simulink model "ForwardDyn_CTC_SCARA"  (R2023a)
settings: Solver=FixedStepAuto  StartTime=0.0  StopTime=10  FixedStep=0.01  RelTol=1e-3
libraries: slpidlib x4
settings Model: Creator=abdom  LastModifiedBy=abdom

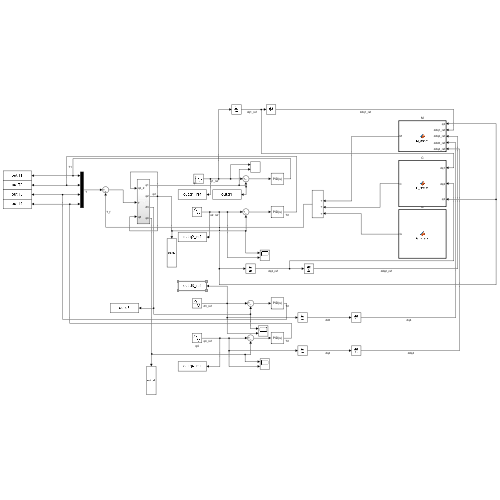
[thumbnail: Simulink's stored preview of the top-level diagram]
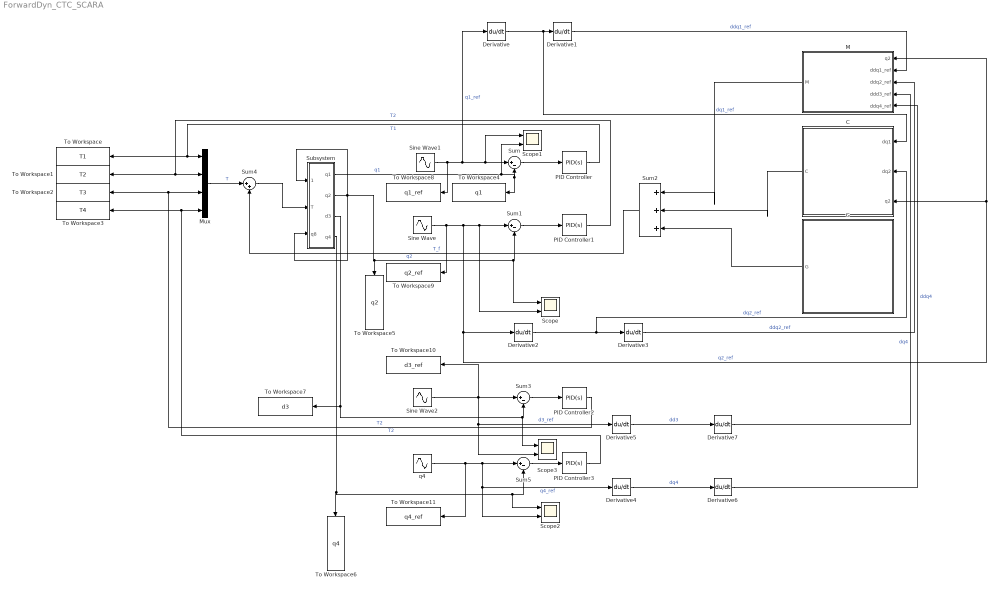
== system ForwardDyn_CTC_SCARA ==
  C : MATLAB Function  TreatAsAtomicUnit=on
  Derivative{,1..7} (8 alike) : Derivative
  G : MATLAB Function  TreatAsAtomicUnit=on
  M : MATLAB Function  TreatAsAtomicUnit=on
  Mux : Mux
  PID Controller : slpidlib/PID Controller  Controller=PID  Form=Parallel  TimeDomain=Continuous-time  UseExternalTs=off  SampleTime=-1  IntegratorMethod=Forward Euler  FilterMethod=Forward Euler  ControllerParametersSource=internal  P=100  I=70  UseKiTs=off  D=10  N=100  UseFilter=on  TunerSelectOption=Transfer Function Based (PID Tuner App)  InitialConditionSource=internal  InitialConditionForIntegrator=0  InitialConditionForFilter=0  DifferentiatorICPrevScaledInput=0  ExternalReset=none  TrackingMode=off  Kt=1  LimitOutput=off  SatLimitsSource=internal  UpperSaturationLimit=inf  LowerSaturationLimit=-inf  LinearizeAsGain=on  AntiWindupMode=none  Kb=1  LimitIntegrator=off  UpperIntegratorSaturationLimit=inf  LowerIntegratorSaturationLimit=-inf  POutMin=[]  POutMax=[]  IOutMin=[]  IOutMax=[]  DOutMin=[]  DOutMax=[]  NOutMin=[]  NOutMax=[]  SumOutMin=[]  SumOutMax=[]  SaturationOutMin=[]  SaturationOutMax=[]  PParamMin=[]  PParamMax=[]  IParamMin=[]  IParamMax=[]  DParamMin=[]  DParamMax=[]  NParamMin=[]  NParamMax=[]  KbParamMin=[]  KbParamMax=[]  KtParamMin=[]  KtParamMax=[]  KbOutMin=[]  KbOutMax=[]  KtOutMin=[]  KtOutMax=[]  IntegratorOutMin=[]  IntegratorOutMax=[]  FilterOutMin=[]  FilterOutMax=[]  SumI1OutMin=[]  SumI1OutMax=[]  SumI2OutMin=[]  SumI2OutMax=[]  SumI3OutMin=[]  SumI3OutMax=[]  SumI4OutMin=[]  SumI4OutMax=[]  SumDOutMin=[]  SumDOutMax=[]  DifferentiatorOutMin=[]  DifferentiatorOutMax=[]  FilterDiffOutCoefMin=[]  FilterDiffOutCoefMax=[]  ReciprocalOutMin=[]  ReciprocalOutMax=[]  SumDenOutMin=[]  SumDenOutMax=[]  SumNumOutMin=[]  SumNumOutMax=[]  DivideOutMin=[]  DivideOutMax=[]  UdiffTsProdOutMin=[]  UdiffTsProdOutMax=[]  NTsProdOutMin=[]  NTsProdOutMax=[]  UintegralTsProdOutMin=[]  UintegralTsProdOutMax=[]  UngainTsProdOutMin=[]  UngainTsProdOutMax=[]  ClampingZeroOutDataTypeStr=Inherit: Inherit via back propagation  ClampingZeroOutMin=[]  ClampingZeroOutMax=[]  FilterDenConstantOutDataTypeStr=Inherit: Inherit via back propagation  FilterDenConstantOutMin=[]  FilterDenConstantOutMax=[]  PCopyOutDataTypeStr=Inherit: Inherit via back propagation  PCopyOutMin=[]  PCopyOutMax=[]  NCopyOutDataTypeStr=Inherit: Inherit via back propagation  NCopyOutMin=[]  NCopyOutMax=[]  IntegratorContinuousStateAttributes=''  IntegratorStateMustResolveToSignalObject=off  IntegratorRTWStateStorageClass=Auto  FilterContinuousStateAttributes=''  FilterStateMustResolveToSignalObject=off  FilterRTWStateStorageClass=Auto  ParallelPVariant=InternalParameters  IdealPVariant=Disabled  IVariant=InternalParameters  DVariant=InternalParameters  IntegratorVariant=Continuous  SatVariant=Disabled  AWVariant=Passthrough  PCopyVariant=Disabled  TRVariant=Disabled  FdbkBlocksVariant=Forward  IdealPFdbkVariant=Disabled  SatFdbkVariant=Disabled  DerivativeFilterVariant=ContFilter  NVariant=InternalParameters  NCopyVariant=Disabled  FilterICVariant=InternalICsFilter  IntegratorICVariant=InternalICs  ExternalResetVariant=Disabled  TRSumVariant=Passthrough  SumFdbkVariant=Disabled  SumVariant=Sum_PID  TsampFilterVariant=InternalTs  TsampNgainVariant=Passthrough  TsampIntegralVariant=Disabled_SignalSpec  ExternalSaturationOutDataTypeStr=Inherit: Same as second input
  PID Controller1 : slpidlib/PID Controller  Controller=PID  Form=Parallel  TimeDomain=Continuous-time  UseExternalTs=off  SampleTime=-1  IntegratorMethod=Forward Euler  FilterMethod=Forward Euler  ControllerParametersSource=internal  P=100  I=30  UseKiTs=off  D=10  N=1  UseFilter=on  TunerSelectOption=Transfer Function Based (PID Tuner App)  InitialConditionSource=internal  InitialConditionForIntegrator=0  InitialConditionForFilter=0  DifferentiatorICPrevScaledInput=0  ExternalReset=none  TrackingMode=off  Kt=1  LimitOutput=off  SatLimitsSource=internal  UpperSaturationLimit=inf  LowerSaturationLimit=-inf  LinearizeAsGain=on  AntiWindupMode=none  Kb=1  LimitIntegrator=off  UpperIntegratorSaturationLimit=inf  LowerIntegratorSaturationLimit=-inf  POutMin=[]  POutMax=[]  IOutMin=[]  IOutMax=[]  DOutMin=[]  DOutMax=[]  NOutMin=[]  NOutMax=[]  SumOutMin=[]  SumOutMax=[]  SaturationOutMin=[]  SaturationOutMax=[]  PParamMin=[]  PParamMax=[]  IParamMin=[]  IParamMax=[]  DParamMin=[]  DParamMax=[]  NParamMin=[]  NParamMax=[]  KbParamMin=[]  KbParamMax=[]  KtParamMin=[]  KtParamMax=[]  KbOutMin=[]  KbOutMax=[]  KtOutMin=[]  KtOutMax=[]  IntegratorOutMin=[]  IntegratorOutMax=[]  FilterOutMin=[]  FilterOutMax=[]  SumI1OutMin=[]  SumI1OutMax=[]  SumI2OutMin=[]  SumI2OutMax=[]  SumI3OutMin=[]  SumI3OutMax=[]  SumI4OutMin=[]  SumI4OutMax=[]  SumDOutMin=[]  SumDOutMax=[]  DifferentiatorOutMin=[]  DifferentiatorOutMax=[]  FilterDiffOutCoefMin=[]  FilterDiffOutCoefMax=[]  ReciprocalOutMin=[]  ReciprocalOutMax=[]  SumDenOutMin=[]  SumDenOutMax=[]  SumNumOutMin=[]  SumNumOutMax=[]  DivideOutMin=[]  DivideOutMax=[]  UdiffTsProdOutMin=[]  UdiffTsProdOutMax=[]  NTsProdOutMin=[]  NTsProdOutMax=[]  UintegralTsProdOutMin=[]  UintegralTsProdOutMax=[]  UngainTsProdOutMin=[]  UngainTsProdOutMax=[]  ClampingZeroOutDataTypeStr=Inherit: Inherit via back propagation  ClampingZeroOutMin=[]  ClampingZeroOutMax=[]  FilterDenConstantOutDataTypeStr=Inherit: Inherit via back propagation  FilterDenConstantOutMin=[]  FilterDenConstantOutMax=[]  PCopyOutDataTypeStr=Inherit: Inherit via back propagation  PCopyOutMin=[]  PCopyOutMax=[]  NCopyOutDataTypeStr=Inherit: Inherit via back propagation  NCopyOutMin=[]  NCopyOutMax=[]  IntegratorContinuousStateAttributes=''  IntegratorStateMustResolveToSignalObject=off  IntegratorRTWStateStorageClass=Auto  FilterContinuousStateAttributes=''  FilterStateMustResolveToSignalObject=off  FilterRTWStateStorageClass=Auto  ParallelPVariant=InternalParameters  IdealPVariant=Disabled  IVariant=InternalParameters  DVariant=InternalParameters  IntegratorVariant=Continuous  SatVariant=Disabled  AWVariant=Passthrough  PCopyVariant=Disabled  TRVariant=Disabled  FdbkBlocksVariant=Forward  IdealPFdbkVariant=Disabled  SatFdbkVariant=Disabled  DerivativeFilterVariant=ContFilter  NVariant=InternalParameters  NCopyVariant=Disabled  FilterICVariant=InternalICsFilter  IntegratorICVariant=InternalICs  ExternalResetVariant=Disabled  TRSumVariant=Passthrough  SumFdbkVariant=Disabled  SumVariant=Sum_PID  TsampFilterVariant=InternalTs  TsampNgainVariant=Passthrough  TsampIntegralVariant=Disabled_SignalSpec  ExternalSaturationOutDataTypeStr=Inherit: Same as second input
  PID Controller2 : slpidlib/PID Controller  Controller=PID  Form=Parallel  TimeDomain=Continuous-time  UseExternalTs=off  SampleTime=-1  IntegratorMethod=Forward Euler  FilterMethod=Forward Euler  ControllerParametersSource=internal  P=150  I=50  UseKiTs=off  D=5  N=1  UseFilter=on  TunerSelectOption=Transfer Function Based (PID Tuner App)  InitialConditionSource=internal  InitialConditionForIntegrator=0  InitialConditionForFilter=0  DifferentiatorICPrevScaledInput=0  ExternalReset=none  TrackingMode=off  Kt=1  LimitOutput=off  SatLimitsSource=internal  UpperSaturationLimit=inf  LowerSaturationLimit=-inf  LinearizeAsGain=on  AntiWindupMode=none  Kb=1  LimitIntegrator=off  UpperIntegratorSaturationLimit=inf  LowerIntegratorSaturationLimit=-inf  POutMin=[]  POutMax=[]  IOutMin=[]  IOutMax=[]  DOutMin=[]  DOutMax=[]  NOutMin=[]  NOutMax=[]  SumOutMin=[]  SumOutMax=[]  SaturationOutMin=[]  SaturationOutMax=[]  PParamMin=[]  PParamMax=[]  IParamMin=[]  IParamMax=[]  DParamMin=[]  DParamMax=[]  NParamMin=[]  NParamMax=[]  KbParamMin=[]  KbParamMax=[]  KtParamMin=[]  KtParamMax=[]  KbOutMin=[]  KbOutMax=[]  KtOutMin=[]  KtOutMax=[]  IntegratorOutMin=[]  IntegratorOutMax=[]  FilterOutMin=[]  FilterOutMax=[]  SumI1OutMin=[]  SumI1OutMax=[]  SumI2OutMin=[]  SumI2OutMax=[]  SumI3OutMin=[]  SumI3OutMax=[]  SumI4OutMin=[]  SumI4OutMax=[]  SumDOutMin=[]  SumDOutMax=[]  DifferentiatorOutMin=[]  DifferentiatorOutMax=[]  FilterDiffOutCoefMin=[]  FilterDiffOutCoefMax=[]  ReciprocalOutMin=[]  ReciprocalOutMax=[]  SumDenOutMin=[]  SumDenOutMax=[]  SumNumOutMin=[]  SumNumOutMax=[]  DivideOutMin=[]  DivideOutMax=[]  UdiffTsProdOutMin=[]  UdiffTsProdOutMax=[]  NTsProdOutMin=[]  NTsProdOutMax=[]  UintegralTsProdOutMin=[]  UintegralTsProdOutMax=[]  UngainTsProdOutMin=[]  UngainTsProdOutMax=[]  ClampingZeroOutDataTypeStr=Inherit: Inherit via back propagation  ClampingZeroOutMin=[]  ClampingZeroOutMax=[]  FilterDenConstantOutDataTypeStr=Inherit: Inherit via back propagation  FilterDenConstantOutMin=[]  FilterDenConstantOutMax=[]  PCopyOutDataTypeStr=Inherit: Inherit via back propagation  PCopyOutMin=[]  PCopyOutMax=[]  NCopyOutDataTypeStr=Inherit: Inherit via back propagation  NCopyOutMin=[]  NCopyOutMax=[]  IntegratorContinuousStateAttributes=''  IntegratorStateMustResolveToSignalObject=off  IntegratorRTWStateStorageClass=Auto  FilterContinuousStateAttributes=''  FilterStateMustResolveToSignalObject=off  FilterRTWStateStorageClass=Auto  ParallelPVariant=InternalParameters  IdealPVariant=Disabled  IVariant=InternalParameters  DVariant=InternalParameters  IntegratorVariant=Continuous  SatVariant=Disabled  AWVariant=Passthrough  PCopyVariant=Disabled  TRVariant=Disabled  FdbkBlocksVariant=Forward  IdealPFdbkVariant=Disabled  SatFdbkVariant=Disabled  DerivativeFilterVariant=ContFilter  NVariant=InternalParameters  NCopyVariant=Disabled  FilterICVariant=InternalICsFilter  IntegratorICVariant=InternalICs  ExternalResetVariant=Disabled  TRSumVariant=Passthrough  SumFdbkVariant=Disabled  SumVariant=Sum_PID  TsampFilterVariant=InternalTs  TsampNgainVariant=Passthrough  TsampIntegralVariant=Disabled_SignalSpec  ExternalSaturationOutDataTypeStr=Inherit: Same as second input
  PID Controller3 : slpidlib/PID Controller  Controller=PID  Form=Parallel  TimeDomain=Continuous-time  UseExternalTs=off  SampleTime=-1  IntegratorMethod=Forward Euler  FilterMethod=Forward Euler  ControllerParametersSource=internal  P=100  I=30  UseKiTs=off  D=10  N=1  UseFilter=on  TunerSelectOption=Transfer Function Based (PID Tuner App)  InitialConditionSource=internal  InitialConditionForIntegrator=0  InitialConditionForFilter=0  DifferentiatorICPrevScaledInput=0  ExternalReset=none  TrackingMode=off  Kt=1  LimitOutput=off  SatLimitsSource=internal  UpperSaturationLimit=inf  LowerSaturationLimit=-inf  LinearizeAsGain=on  AntiWindupMode=none  Kb=1  LimitIntegrator=off  UpperIntegratorSaturationLimit=inf  LowerIntegratorSaturationLimit=-inf  POutMin=[]  POutMax=[]  IOutMin=[]  IOutMax=[]  DOutMin=[]  DOutMax=[]  NOutMin=[]  NOutMax=[]  SumOutMin=[]  SumOutMax=[]  SaturationOutMin=[]  SaturationOutMax=[]  PParamMin=[]  PParamMax=[]  IParamMin=[]  IParamMax=[]  DParamMin=[]  DParamMax=[]  NParamMin=[]  NParamMax=[]  KbParamMin=[]  KbParamMax=[]  KtParamMin=[]  KtParamMax=[]  KbOutMin=[]  KbOutMax=[]  KtOutMin=[]  KtOutMax=[]  IntegratorOutMin=[]  IntegratorOutMax=[]  FilterOutMin=[]  FilterOutMax=[]  SumI1OutMin=[]  SumI1OutMax=[]  SumI2OutMin=[]  SumI2OutMax=[]  SumI3OutMin=[]  SumI3OutMax=[]  SumI4OutMin=[]  SumI4OutMax=[]  SumDOutMin=[]  SumDOutMax=[]  DifferentiatorOutMin=[]  DifferentiatorOutMax=[]  FilterDiffOutCoefMin=[]  FilterDiffOutCoefMax=[]  ReciprocalOutMin=[]  ReciprocalOutMax=[]  SumDenOutMin=[]  SumDenOutMax=[]  SumNumOutMin=[]  SumNumOutMax=[]  DivideOutMin=[]  DivideOutMax=[]  UdiffTsProdOutMin=[]  UdiffTsProdOutMax=[]  NTsProdOutMin=[]  NTsProdOutMax=[]  UintegralTsProdOutMin=[]  UintegralTsProdOutMax=[]  UngainTsProdOutMin=[]  UngainTsProdOutMax=[]  ClampingZeroOutDataTypeStr=Inherit: Inherit via back propagation  ClampingZeroOutMin=[]  ClampingZeroOutMax=[]  FilterDenConstantOutDataTypeStr=Inherit: Inherit via back propagation  FilterDenConstantOutMin=[]  FilterDenConstantOutMax=[]  PCopyOutDataTypeStr=Inherit: Inherit via back propagation  PCopyOutMin=[]  PCopyOutMax=[]  NCopyOutDataTypeStr=Inherit: Inherit via back propagation  NCopyOutMin=[]  NCopyOutMax=[]  IntegratorContinuousStateAttributes=''  IntegratorStateMustResolveToSignalObject=off  IntegratorRTWStateStorageClass=Auto  FilterContinuousStateAttributes=''  FilterStateMustResolveToSignalObject=off  FilterRTWStateStorageClass=Auto  ParallelPVariant=InternalParameters  IdealPVariant=Disabled  IVariant=InternalParameters  DVariant=InternalParameters  IntegratorVariant=Continuous  SatVariant=Disabled  AWVariant=Passthrough  PCopyVariant=Disabled  TRVariant=Disabled  FdbkBlocksVariant=Forward  IdealPFdbkVariant=Disabled  SatFdbkVariant=Disabled  DerivativeFilterVariant=ContFilter  NVariant=InternalParameters  NCopyVariant=Disabled  FilterICVariant=InternalICsFilter  IntegratorICVariant=InternalICs  ExternalResetVariant=Disabled  TRSumVariant=Passthrough  SumFdbkVariant=Disabled  SumVariant=Sum_PID  TsampFilterVariant=InternalTs  TsampNgainVariant=Passthrough  TsampIntegralVariant=Disabled_SignalSpec  ExternalSaturationOutDataTypeStr=Inherit: Same as second input
  Scope{,1..3} (4 alike) : Scope  NumInputPorts=2
  Sine Wave : Sin  SampleTime=0
  Sine Wave1 : Sin  SampleTime=0
  Sine Wave2 : Sin  Amplitude=0.05  Frequency=0.5  SampleTime=0
  Subsystem : Subsystem
  Sum{,1,3,5} (4 alike) : Sum  Inputs=|+-
  Sum2 : Sum  Inputs=|+++
  Sum4 : Sum  Inputs=|++
  To Workspace : ToWorkspace  VariableName=T1  SampleTime=-1
  To Workspace1 : ToWorkspace  VariableName=T2  SampleTime=-1
  To Workspace10 : ToWorkspace  VariableName=d3_ref  SampleTime=-1
  To Workspace11 : ToWorkspace  VariableName=q4_ref  SampleTime=-1
  To Workspace2 : ToWorkspace  VariableName=T3  SampleTime=-1
  To Workspace3 : ToWorkspace  VariableName=T4  SampleTime=-1
  To Workspace4 : ToWorkspace  VariableName=q1  SampleTime=-1
  To Workspace5 : ToWorkspace  VariableName=q2  SampleTime=-1
  To Workspace6 : ToWorkspace  VariableName=q4  SampleTime=-1
  To Workspace7 : ToWorkspace  VariableName=d3  SampleTime=-1
  To Workspace8 : ToWorkspace  VariableName=q1_ref  SampleTime=-1
  To Workspace9 : ToWorkspace  VariableName=q2_ref  SampleTime=-1
  q4 : Sin  SampleTime=0
  wires:
  PID Controller/1 -> To Workspace/1, Mux/1  "T1"
  Subsystem/1(q1) -> To Workspace4/1, Sum/2, Scope1/2  "q1"
  Subsystem/2(q2) -> Subsystem/3(q8), Scope/1, Sum1/2, To Workspace5/1, Subsystem/1(q2_2)  "q2"
  Sine Wave1/1 -> To Workspace8/1, Derivative/1, Scope1/1, Sum/1  "q1_ref"
  Sine Wave/1 -> To Workspace9/1, C/3(q2), M/1(q2), Derivative2/1, Scope/2, Sum1/1  "q2_ref"
  Sum/1 -> PID Controller/1
  Sum1/1 -> PID Controller1/1
  PID Controller1/1 -> Mux/2, To Workspace1/1  "T2"
  Derivative/1 -> C/1(dq1), Derivative1/1  "dq1_ref"
  Derivative1/1 -> M/2(ddq1_ref)  "ddq1_ref"
  Derivative2/1 -> C/2(dq2), Derivative3/1  "dq2_ref"
  Derivative3/1 -> M/3(ddq2_ref)  "ddq2_ref"
  Mux/1 -> Sum4/1  "T"
  Sum2/1 -> Sum4/2  "T_f"
  Sum4/1 -> Subsystem/2(T)
  M/1(M) -> Sum2/1
  G/1(G) -> Sum2/3
  C/1(C) -> Sum2/2
  Subsystem/3(d3) -> To Workspace7/1, Scope3/1, Sum3/2
  Subsystem/4(q4) -> To Workspace6/1, Scope2/1, Sum5/2
  q4/1 -> To Workspace11/1, Scope2/2, Derivative4/1, Sum5/1  "q4_ref"
  Sine Wave2/1 -> To Workspace10/1, Scope3/2, Derivative5/1, Sum3/1  "d3_ref"
  Sum3/1 -> PID Controller2/1
  Sum5/1 -> PID Controller3/1
  PID Controller2/1 -> Mux/3, To Workspace2/1  "T2"
  PID Controller3/1 -> Mux/4, To Workspace3/1  "T2"
  Derivative5/1 -> Derivative7/1  "dd3"
  Derivative4/1 -> Derivative6/1  "dq4"
  Derivative7/1 -> M/4(ddd3_ref)  "dq4"
  Derivative6/1 -> M/5(ddq4_ref)  "ddq4"

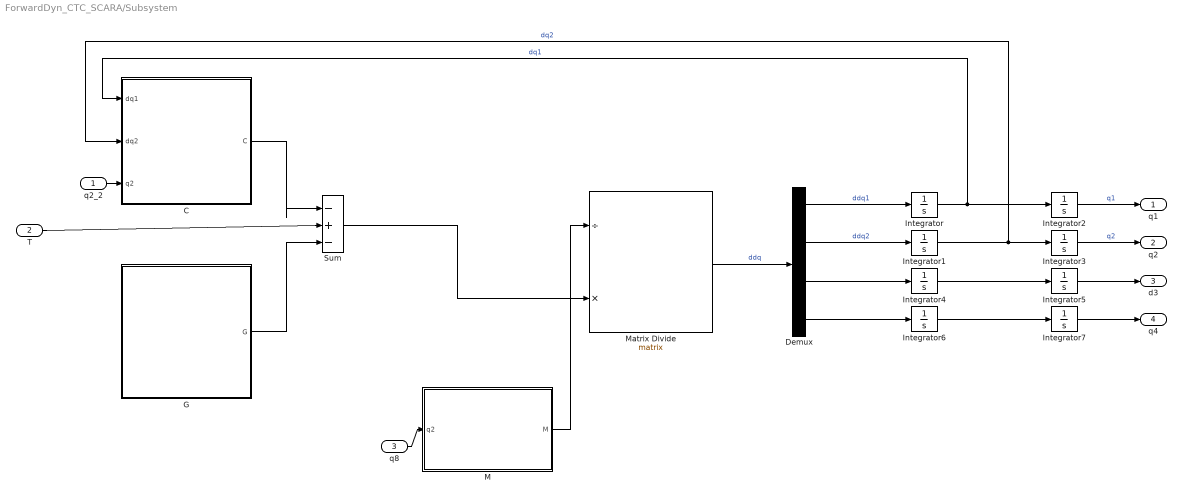
== system ForwardDyn_CTC_SCARA/Subsystem ==
  q2_2 : Inport
  T : Inport  Port=2
  q8 : Inport  Port=3
  C : MATLAB Function  TreatAsAtomicUnit=on
  Demux : Demux
  G : MATLAB Function  TreatAsAtomicUnit=on
  Integrator{,1..7} (8 alike) : Integrator
  M : MATLAB Function  TreatAsAtomicUnit=on
  Matrix Divide : Product  Inputs=/*  Multiplication=Matrix(*)
  Sum : Sum  Inputs=|-+-
  q1 : Outport
  q2 : Outport  Port=2
  d3 : Outport  Port=3
  q4 : Outport  Port=4
  wires:
  G/1(G) -> Sum/3
  Matrix Divide/1 -> Demux/1  "ddq"
  Integrator1/1 -> C/2(dq2), Integrator3/1  "dq2"
  Integrator/1 -> C/1(dq1), Integrator2/1  "dq1"
  Sum/1 -> Matrix Divide/2
  C/1(C) -> Sum/1
  T/1 -> Sum/2
  Demux/1 -> Integrator/1  "ddq1"
  Demux/2 -> Integrator1/1  "ddq2"
  q8/1 -> M/1(q2)
  M/1(M) -> Matrix Divide/1
  Integrator2/1 -> q1/1  "q1"
  q2_2/1 -> C/3(q2)
  Integrator3/1 -> q2/1  "q2"
  Demux/3 -> Integrator4/1
  Integrator4/1 -> Integrator5/1
  Integrator5/1 -> d3/1
  Integrator7/1 -> q4/1
  Integrator6/1 -> Integrator7/1
  Demux/4 -> Integrator6/1

== matlab function ForwardDyn_CTC_SCARA/Subsystem/C ==
  data: dq1 input; C output; dq2 input; q2 input
function C = C_scara(dq1,dq2,q2)
%C_scara
%    C = C_scara(L2,L3,DQ1,DQ2,M2,M3,M4,Q2)

%    This function was generated by the Symbolic Math Toolbox version 9.3.
%    12-May-2025 16:21:30
L2 = 0.6;
L3 = 0.4;
m2 = 3.0;
m3 = 2.5;
m4 = 1.0;


t2 = sin(q2);
t3 = m3.*2.0;
t4 = m4.*2.0;
t5 = m2+t3+t4;
C = [L2.*L3.*dq2.*t2.*t5.*(dq1.*2.0+dq2).*(-1.0./2.0);(L2.*L3.*dq1.^2.*t2.*t5)./2.0;0.0;0.0];
end

== matlab function ForwardDyn_CTC_SCARA/Subsystem/M ==
  data: M output; q2 input
function M = M_scara(q2)
%M_scara
%    M = M_scara(Izz1,Izz2,Izz4,L2,L3,M1,M2,M3,M4,Q2)

%    This function was generated by the Symbolic Math Toolbox version 9.3.
%    12-May-2025 16:21:29


L2 = 0.6;
L3 = 0.4;
m1 = 5.0;
m2 = 3.0;
m3 = 2.5;
m4 = 1.0;
Izz1 = 0.20;
Izz2 = 0.08;
Izz4 = 0.02;


t2 = cos(q2);
t3 = L2.^2;
t4 = L3.^2;
t5 = m3.*t4;
t6 = m4.*t4;
t7 = L2.*L3.*m3.*t2;
t8 = L2.*L3.*m4.*t2;
t9 = (m2.*t4)./4.0;
t10 = (L2.*L3.*m2.*t2)./2.0;
t11 = Izz2+Izz4+t5+t6+t7+t8+t9+t10;
M = reshape([Izz1+Izz2+Izz4+t5+t6+t7.*2.0+t8.*2.0+t9+(m1.*t3)./4.0+m2.*t3+m3.*t3+m4.*t3+L2.*L3.*m2.*t2,t11,0.0,Izz4,t11,Izz2+Izz4+t5+t6+t9,0.0,Izz4,0.0,0.0,m3./4.0+m4,0.0,Izz4,Izz4,0.0,Izz4],[4,4]);
end

== matlab function ForwardDyn_CTC_SCARA/Subsystem/G ==
  data: G output
function G = G_scara()
%G_scara
%    G = G_scara(M3,M4)

%    This function was generated by the Symbolic Math Toolbox version 9.3.
%    12-May-2025 16:21:30

m3 = 2.5;
m4 = 1.0;


G = [0.0;0.0;m3.*(9.81e+2./2.0e+2)+m4.*(9.81e+2./1.0e+2);0.0];
end

== matlab function ForwardDyn_CTC_SCARA/G ==
  data: G output
function G = G_scara()
%G_scara
%    G = G_scara(M3,M4)

%    This function was generated by the Symbolic Math Toolbox version 9.3.
%    12-May-2025 16:21:30

m3 = 2.5;
m4 = 1.0;


G = [0.0;0.0;m3.*(9.81e+2./2.0e+2)+m4.*(9.81e+2./1.0e+2);0.0];
end

== matlab function ForwardDyn_CTC_SCARA/C ==
  data: dq1 input; C output; dq2 input; q2 input
function C = C_scara(dq1,dq2,q2)
%C_scara
%    C = C_scara(L2,L3,DQ1,DQ2,M2,M3,M4,Q2)

%    This function was generated by the Symbolic Math Toolbox version 9.3.
%    12-May-2025 16:21:30
L2 = 0.6;
L3 = 0.4;
m2 = 3.0;
m3 = 2.5;
m4 = 1.0;


t2 = sin(q2);
t3 = m3.*2.0;
t4 = m4.*2.0;
t5 = m2+t3+t4;
C = [L2.*L3.*dq2.*t2.*t5.*(dq1.*2.0+dq2).*(-1.0./2.0);(L2.*L3.*dq1.^2.*t2.*t5)./2.0;0.0;0.0];
end

== matlab function ForwardDyn_CTC_SCARA/M ==
  data: M output; q2 input; ddq1_ref input; ddq2_ref input; ddd3_ref input; ddq4_ref input
function M = M_scara(q2, ddq1_ref, ddq2_ref, ddd3_ref, ddq4_ref)
%M_scara
%    M = M_scara(Izz1,Izz2,Izz4,L2,L3,M1,M2,M3,M4,Q2)

%    This function was generated by the Symbolic Math Toolbox version 9.3.
%    12-May-2025 16:21:29


L2 = 0.6;
L3 = 0.4;
m1 = 5.0;
m2 = 3.0;
m3 = 2.5;
m4 = 1.0;
Izz1 = 0.20;
Izz2 = 0.08;
Izz4 = 0.02;


t2 = cos(q2);
t3 = L2.^2;
t4 = L3.^2;
t5 = m3.*t4;
t6 = m4.*t4;
t7 = L2.*L3.*m3.*t2;
t8 = L2.*L3.*m4.*t2;
t9 = (m2.*t4)./4.0;
t10 = (L2.*L3.*m2.*t2)./2.0;
t11 = Izz2+Izz4+t5+t6+t7+t8+t9+t10;
M_final = reshape([Izz1+Izz2+Izz4+t5+t6+t7.*2.0+t8.*2.0+t9+(m1.*t3)./4.0+m2.*t3+m3.*t3+m4.*t3+L2.*L3.*m2.*t2,t11,0.0,Izz4,t11,Izz2+Izz4+t5+t6+t9,0.0,Izz4,0.0,0.0,m3./4.0+m4,0.0,Izz4,Izz4,0.0,Izz4],[4,4]);
M = M_final * [ddq1_ref ddq2_ref ddd3_ref ddq4_ref]'; 
end
